simulink model "EvitaParedes_IR"  (R2023b)
settings: Solver=VariableStepAuto  StartTime=0.0  StopTime=10.0  RelTol=1e-3
settings Model: Creator=Usuario_UMA  LastModifiedBy=javie

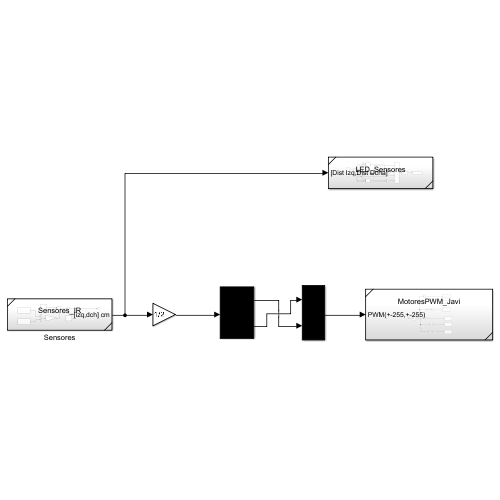
[thumbnail: Simulink's stored preview of the top-level diagram]
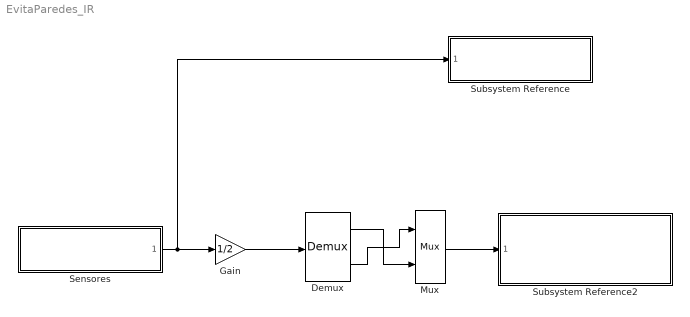
== system EvitaParedes_IR ==
  Demux : Demux  Outputs=2
  Gain : Gain  Gain=1/2
  Mux : Mux  Inputs=2
  Sensores : Subsystem  ReferencedSubsystem=Sensores_IR
  Subsystem Reference : Subsystem  ReferencedSubsystem=LED_Sensores
  Subsystem Reference2 : Subsystem  ReferencedSubsystem=MotoresPWM_Javi
  wires:
  Mux/1 -> Subsystem Reference2/1
  Sensores/1 -> Gain/1, Subsystem Reference/1
  Demux/1 -> Mux/2
  Demux/2 -> Mux/1
  Gain/1 -> Demux/1
